simulink model "AMFC_Quad_New_01_VelEst_01"  (R2017b)
settings: Solver=ode45  StartTime=0.0  StopTime=360  RelTol=1e-3  EnableMultiTasking=on
InitFcn:
  | Cons_AMFC_Quad_New_01
values from neighbouring files (symbols this model uses):
  alpha_Slid = 0.01    [Cons_AMFC_Quad_New_01.m]    (also in Const_Vel_Est_02.m)
  B = 1e+0*eye(n)    [Cons_AMFC_Quad_New_01.m]    (also in Const_Vel_Est_02.m = 1e0*eye(n); constant_Rev01_4Agents_10.m = 1e0*eye(n); constant_Rev01_4Agents_9.m = 1e0*eye(n))
  BBT_inv = ((B'*B)^(-1))*B'    [Cons_AMFC_Quad_New_01.m]    (also in Const_Vel_Est_02.m; constant_Rev01_4Agents_10.m; constant_Rev01_4Agents_9.m)
  gamma_0 = 1e-0*diag([1e-3*ones(3,1);1e-0*ones(3,1)])    [Cons_AMFC_Quad_New_01.m]    (also in Const_Vel_Est_02.m = 1e-1*diag([1e-3*ones(3,1);1e-0*ones(3,1)]); constant_Rev01_4Agents_10.m = 1e+1*diag([1e-3*ones(3,1);1e-0*ones(3,1)]); constant_Rev01_4Agents_9.m = 1e+1*diag([1e-3*ones(6,1);1e-0*ones(6,1)]))
  gamma_1 = 1e+2*diag([1e-3*ones(3,1);1e-0*ones(3,1)])    [Cons_AMFC_Quad_New_01.m]    (also in Const_Vel_Est_02.m; constant_Rev01_4Agents_10.m = 1e+3*diag([1e-3*ones(3,1);1e0*ones(3,1)]); constant_Rev01_4Agents_9.m = 1e+3*diag([1e-3*ones(6,1);1e0*ones(6,1)]))
  ge = 9.81    [Cons_AMFC_Quad_New_01.m]
  J = 1.2416e-3 * diag([1 1 2])    [Cons_AMFC_Quad_New_01.m]    (also in Const_Vel_Est_02.m = 1.2416e-3 * diag([1 1 2],0); constant_Rev01_4Agents_10.m = 1.2416e-3 * diag([1 1 2],0); constant_Rev01_4Agents_9.m = 1.2416e-3 * diag([1 1 2],0))
  k1 = 10    [Cons_AMFC_Quad_New_01.m]    (also in Const_Vel_Est_02.m = 1; constant_Rev01_4Agents_10.m = 1; constant_Rev01_4Agents_9.m = 1)
  k1o = 1000    [Cons_AMFC_Quad_New_01.m]    (also in Const_Vel_Est_02.m)
  k2 = 0.1    [Cons_AMFC_Quad_New_01.m]    (also in Const_Vel_Est_02.m; constant_Rev01_4Agents_10.m = 1; constant_Rev01_4Agents_9.m = 1)
  k2o = 100    [Cons_AMFC_Quad_New_01.m]    (also in Const_Vel_Est_02.m)
  Ka = 0.01    [Cons_AMFC_Quad_New_01.m]    (also in Const_Vel_Est_02.m; constant_Rev01_4Agents_10.m; constant_Rev01_4Agents_9.m)
  Kd = 0.01    [Cons_AMFC_Quad_New_01.m]    (also in Const_Vel_Est_02.m; constant_Rev01_4Agents_10.m; constant_Rev01_4Agents_9.m)
  Kf = 1.0e-5    (= 1e-05)    [Cons_AMFC_Quad_New_01.m]    (also in Const_Vel_Est_02.m; constant_Rev01_4Agents_10.m; constant_Rev01_4Agents_9.m)
  Kt = 0.0435 * Kf    (= 4.35e-07)    [Cons_AMFC_Quad_New_01.m]    (also in Const_Vel_Est_02.m = 1e-07; constant_Rev01_4Agents_10.m = 1e-07; constant_Rev01_4Agents_9.m = 1e-07)
  L = 0.45    [Cons_AMFC_Quad_New_01.m]    (also in Const_Vel_Est_02.m = DN - AN; constant_Rev01_4Agents_10.m = DN - AN; constant_Rev01_4Agents_9.m = DN - AN)
  m = 6    [Cons_AMFC_Quad_New_01.m]    (also in Const_Vel_Est_02.m; Swing2d_01_const.m = 1)
  M = 2.95    [Cons_AMFC_Quad_New_01.m]    (also in Const_Vel_Est_02.m = 2; constant_Rev01_4Agents_10.m = 2; constant_Rev01_4Agents_9.m = 2)
  n = 6    [Cons_AMFC_Quad_New_01.m]    (also in Const_Vel_Est_02.m; constant_Rev01_4Agents_10.m; constant_Rev01_4Agents_9.m = 12)
  Q = 1e-1*eye(n)    [Cons_AMFC_Quad_New_01.m]    (also in Const_Vel_Est_02.m = 1e-2*eye(n); constant_Rev01_4Agents_10.m = 1e-3*eye(n); constant_Rev01_4Agents_9.m = 1e-3*eye(n))
  R = 1e+0*eye(m)    [Cons_AMFC_Quad_New_01.m]    (also in Const_Vel_Est_02.m = 1e-0*eye(n); constant_Rev01_4Agents_10.m = 1e-0*eye(n); constant_Rev01_4Agents_9.m = 1e-0*eye(n))
  rho_0 = 1e-1    (= 0.1)    [Cons_AMFC_Quad_New_01.m]    (also in Const_Vel_Est_02.m; constant_Rev01_4Agents_10.m = 10; constant_Rev01_4Agents_9.m = 10)
  rho_1 = 1e-0    (= 1)    [Cons_AMFC_Quad_New_01.m]    (also in Const_Vel_Est_02.m; constant_Rev01_4Agents_10.m = 0.1; constant_Rev01_4Agents_9.m = 0.1)
undefined symbols (not defined in the file or in its folder): sigbuilder_block
settings Model: Creator=hp  LastModifiedBy=ali.safaei
settings DataIOCC: LimitDataPoints=on  SaveFormat=Array
settings OptimizationCC: LifeSpan=inf
settings DebuggingCC: UnderspecifiedInitializationDetection=Classic  MergeDetectMultiDrivingBlocksExec=none  SolverPrmCheckMsg=warning  SFUnexpectedBacktrackingDiag=warning  SFNoUnconditionalDefaultTransitionDiag=warning  SFExecutionAtInitializationDiag=none
settings HardwareCC: ProdBitPerPointer=32  ProdBitPerSizeT=32  ProdBitPerPtrDiffT=32  ProdLargestAtomicFloat=None  ProdIntDivRoundTo=Undefined  ProdEndianess=Unspecified  ProdWordSize=32  ProdHWDeviceType=32-bit Generic
settings ModelReferenceCC: PropagateSignalLabelsOutOfModel=off
settings CodeAppCC: StateflowObjectComments=on
settings GRTTargetCC: TargetLangStandard=C89/C90 (ANSI)  GeneratePreprocessorConditionals=Disable all
settings ConfigComp: CovMetricSettings=dw  CovHtmlReporting=on  CovSaveCumulativeToWorkspaceVar=on  CovSaveSingleToWorkspaceVar=on  CovExternalEMLEnable=off

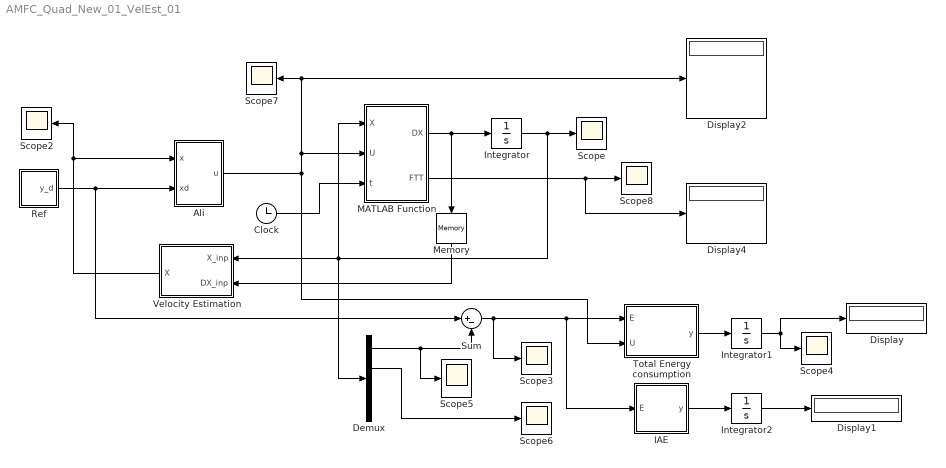
== system AMFC_Quad_New_01_VelEst_01 ==
  Ali : Subsystem
  Clock : Clock
  Demux : Demux
  Display{,1..2,4} (4 alike) : Display
  IAE : MATLAB Function  TreatAsAtomicUnit=on
  Integrator : Integrator  InitialCondition=zeros(12,1)
  Integrator1 : Integrator
  Integrator2 : Integrator
  MATLAB Function : MATLAB Function  TreatAsAtomicUnit=on
  Memory : Memory  InitialCondition=zeros(12,1)
  Ref : Subsystem
  Scope{,2..8} (8 alike) : Scope
  Sum : Sum  Inputs=|+-
  Total Energy consumption : MATLAB Function  TreatAsAtomicUnit=on
  Velocity Estimation : Subsystem
  wires:
  MATLAB Function/1(DX) -> Memory/1, Integrator/1
  Integrator/1 -> Scope/1, Demux/1, MATLAB Function/1(X), Velocity Estimation/1(X_inp)
  Integrator1/1 -> Display/1, Scope4/1
  Total Energy consumption/1(y) -> Integrator1/1
  Ref/1(y_d) -> Sum/1, Ali/2(xd)
  Integrator2/1 -> Display1/1
  Sum/1 -> Total Energy consumption/1(E), IAE/1(E), Scope3/1
  IAE/1(y) -> Integrator2/1
  Demux/1 -> Sum/2, Scope5/1
  Clock/1 -> MATLAB Function/3(t)
  Demux/2 -> Scope6/1
  Ali/1(u) -> Total Energy consumption/2(U), MATLAB Function/2(U), Display2/1, Scope7/1
  MATLAB Function/2(FTT) -> Scope8/1, Display4/1
  Velocity Estimation/1(X) -> Scope2/1, Ali/1(x)
  Memory/1 -> Velocity Estimation/2(DX_inp)

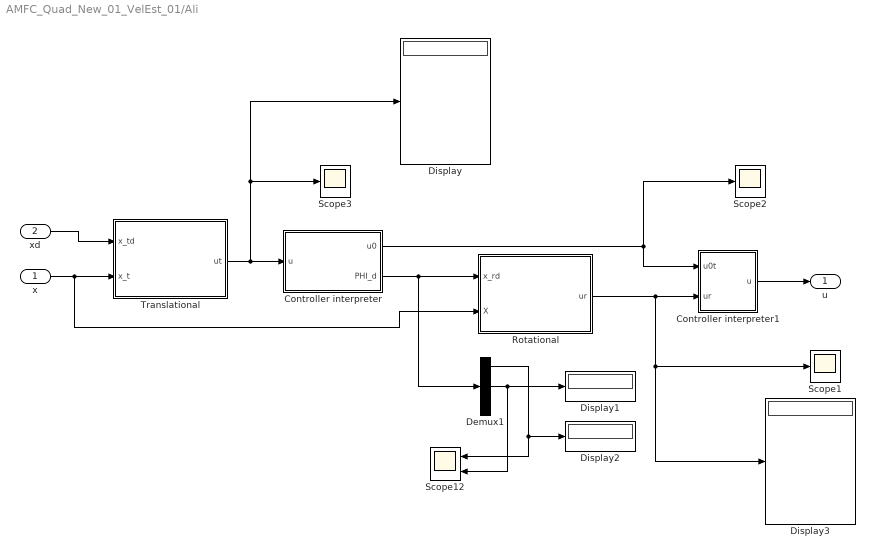
== system AMFC_Quad_New_01_VelEst_01/Ali ==
  x : Inport
  xd : Inport  Port=2
  Controller interpreter : MATLAB Function  TreatAsAtomicUnit=on
  Controller interpreter1 : MATLAB Function  TreatAsAtomicUnit=on
  Demux1 : Demux  Outputs=3
  Display{,1..3} (4 alike) : Display
  Rotational : Subsystem
  Scope1 : Scope
  Scope12 : Scope  NumInputPorts=2
  Scope2 : Scope
  Scope3 : Scope
  Translational : Subsystem
  u : Outport
  wires:
  Controller interpreter/2(PHI_d) -> Demux1/1, Rotational/1(x_rd)
  Rotational/1(ur) -> Display3/1, Scope1/1, Controller interpreter1/2(ur)
  Controller interpreter1/1(u) -> u/1
  Controller interpreter/1(u0) -> Scope2/1, Controller interpreter1/1(u0t)
  Demux1/2 -> Scope12/2, Display1/1
  Demux1/1 -> Display2/1, Scope12/1
  xd/1 -> Translational/1(x_td)
  x/1 -> Rotational/2(X), Translational/2(x_t)
  Translational/1(ut) -> Display/1, Scope3/1, Controller interpreter/1(u)

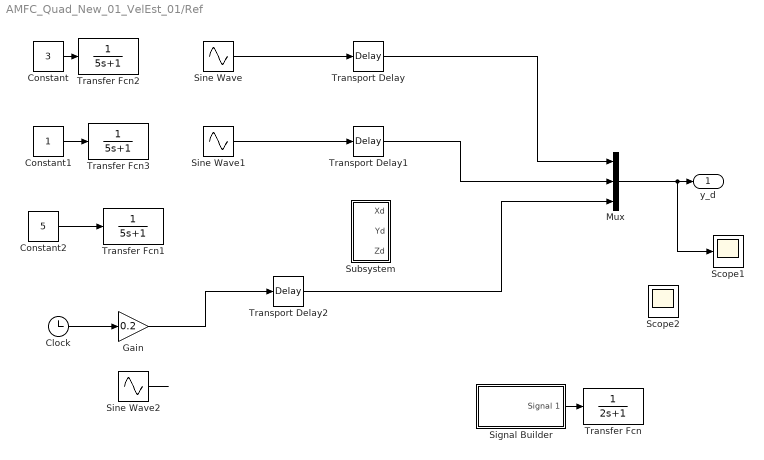
== system AMFC_Quad_New_01_VelEst_01/Ref ==
  Clock : Clock
  Constant : Constant  Value=3
  Constant1 : Constant
  Constant2 : Constant  Value=5
  Gain : Gain  Gain=0.2
  Mux : Mux  Inputs=3
  Scope1 : Scope
  Scope2 : Scope
  Signal Builder : Subsystem  Tag=STV Subsys  LoadFcn=sigbuilder_block('load');  StartFcn=sigbuilder_block('start');  StopFcn=sigbuilder_block('stop');  ClipboardFcn=sigbuilder_block('clipboard');  mask(Sigbuilder block){tuvar=[0:10]}
      mask help: Simulink:masks:SigbuilderBlock_MD
      mask init:
      | if ~strcmp(get_param(bdroot(gcbh),'SimulationStatus'),'stopped') tuvar = sigbuilder_block('maskInit'); end
      settings: CopyFcn=sigbuilder_block('copy');  DeleteFcn=sigbuilder_block('delete');  ModelCloseFcn=sigbuilder_block('modelClose');  PreSaveFcn=sigbuilder_block('preSave');  PauseFcn=sigbuilder_block('pause');  ContinueFcn=sigbuilder_block('continue');  NameChangeFcn=sigbuilder_block('namechange');  OpenFcn=sigbuilder_block('open',[437.25 117.75 550.5 394.5 ]);  CloseFcn=sigbuilder_block('close');
      mask Display: plot(0, 0, 100, 100,[2, 2, 32, 32, 2], [68, 8, 8, 68, 68],[32, 2], [38, 38], [32, 19, 2],[53, 60, 44], [32, 17, 17, 2],[16, 16, 31, 31]);txt = getActiveGroup(gcbh);text(2, 100, txt,'verticalAlignment', 'top');
  Sine Wave : Sin  Amplitude=10  Bias=-10  Frequency=0.2  Phase=pi/2  SampleTime=0
  Sine Wave1 : Sin  Amplitude=10  Frequency=0.2  SampleTime=0
  Sine Wave2 : Sin  Amplitude=2  Frequency=0.2  SampleTime=0
  Subsystem : Subsystem
  Transfer Fcn : TransferFcn  Denominator=[2 1]
  Transfer Fcn1 : TransferFcn  Denominator=[5 1]
  Transfer Fcn2 : TransferFcn  Denominator=[5 1]
  Transfer Fcn3 : TransferFcn  Denominator=[5 1]
  Transport Delay : TransportDelay  DelayTime=50
  Transport Delay1 : TransportDelay  DelayTime=50
  Transport Delay2 : TransportDelay  DelayTime=30
  y_d : Outport
  wires:
  Clock/1 -> Gain/1
  Signal Builder/1(Signal 1) -> Transfer Fcn/1
  Mux/1 -> Scope1/1, y_d/1
  Transport Delay/1 -> Mux/1
  Constant2/1 -> Transfer Fcn1/1
  Sine Wave1/1 -> Transport Delay1/1
  Sine Wave/1 -> Transport Delay/1
  Sine Wave2/1 -> ?
  Transport Delay1/1 -> Mux/2
  Constant/1 -> Transfer Fcn2/1
  Constant1/1 -> Transfer Fcn3/1
  Transport Delay2/1 -> Mux/3
  Gain/1 -> Transport Delay2/1

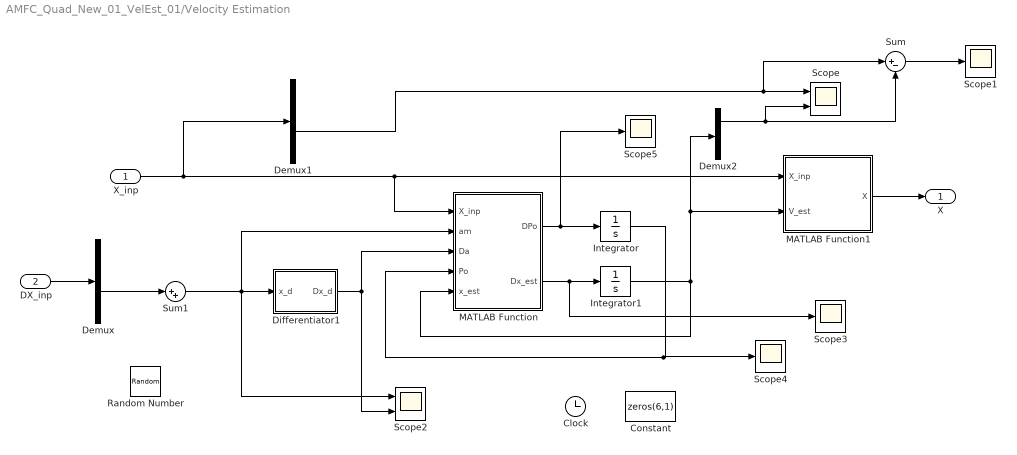
== system AMFC_Quad_New_01_VelEst_01/Velocity Estimation ==
  X_inp : Inport
  DX_inp : Inport  Port=2
  Clock : Clock
  Constant : Constant  Value=zeros(6,1)
  Demux : Demux
  Demux1 : Demux
  Demux2 : Demux  Outputs=2
  Differentiator1 : Subsystem
  Integrator : Integrator  InitialCondition=zeros(6)
  Integrator1 : Integrator  InitialCondition=zeros(6,1)
  MATLAB Function : MATLAB Function  TreatAsAtomicUnit=on
  MATLAB Function1 : MATLAB Function  TreatAsAtomicUnit=on
  Random Number : RandomNumber
  Scope : Scope  NumInputPorts=2
  Scope{1,3..5} (4 alike) : Scope
  Scope2 : Scope  NumInputPorts=2
  Sum : Sum  Inputs=|+-
  Sum1 : Sum  Inputs=|++
  X : Outport
  wires:
  DX_inp/1 -> Demux/1
  X_inp/1 -> Demux1/1, MATLAB Function/1(X_inp), MATLAB Function1/1(X_inp)
  MATLAB Function/1(DPo) -> Scope5/1, Integrator/1
  MATLAB Function/2(Dx_est) -> Integrator1/1, Scope3/1
  MATLAB Function1/1(X) -> X/1
  Differentiator1/1(Dx_d) -> Scope2/2, MATLAB Function/3(Da)
  Demux1/3 -> Sum/1, Scope/1
  Demux2/1 -> Sum/2, Scope/2
  Sum/1 -> Scope1/1
  Demux/3 -> Sum1/1
  Integrator1/1 -> MATLAB Function1/2(V_est), Demux2/1, MATLAB Function/5(x_est)
  Sum1/1 -> MATLAB Function/2(am), Differentiator1/1(x_d), Scope2/1
  Integrator/1 -> Scope4/1, MATLAB Function/4(Po)

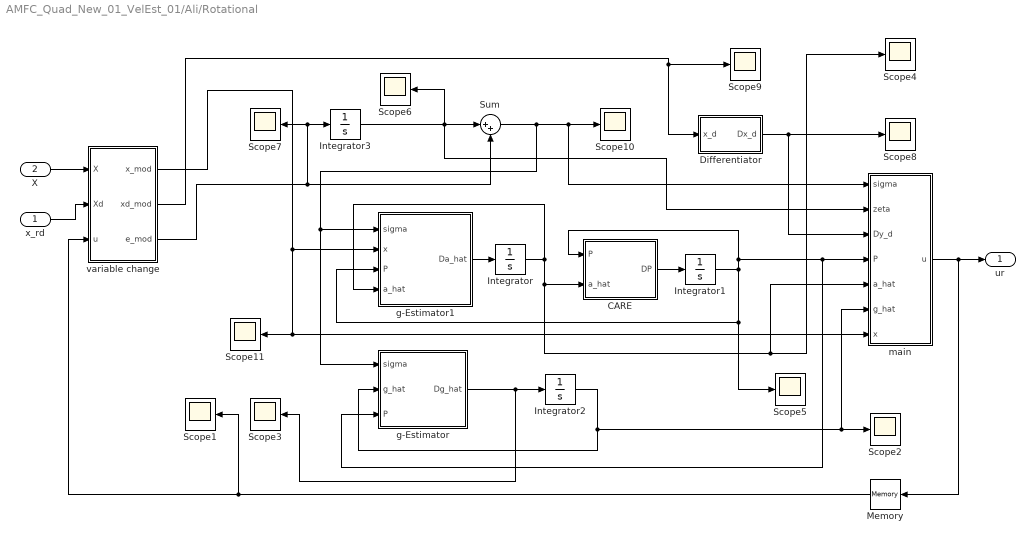
== system AMFC_Quad_New_01_VelEst_01/Ali/Rotational ==
  x_rd : Inport
  X : Inport  Port=2
  CARE : MATLAB Function  TreatAsAtomicUnit=on
  Differentiator : Subsystem
  Integrator : Integrator  InitialCondition=zeros(n)
  Integrator1 : Integrator  InitialCondition=eye(n)
  Integrator2 : Integrator  InitialCondition=zeros(n,1)
  Integrator3 : Integrator  InitialCondition=zeros(n,1)
  Memory : Memory  InitialCondition=zeros(m,1)
  Scope{1..11} (11 alike) : Scope
  Sum : Sum  Inputs=|++
  g-Estimator : MATLAB Function  TreatAsAtomicUnit=on
  g-Estimator1 : MATLAB Function  TreatAsAtomicUnit=on
  main : MATLAB Function  TreatAsAtomicUnit=on
  variable change : MATLAB Function  TreatAsAtomicUnit=on
  ur : Outport
  wires:
  x_rd/1 -> variable change/2(Xd)
  X/1 -> variable change/1(X)
  CARE/1(DP) -> Integrator1/1
  Sum/1 -> main/1(sigma), Scope10/1, g-Estimator/1(sigma), g-Estimator1/1(sigma)
  g-Estimator1/1(Da_hat) -> Integrator/1
  variable change/1(x_mod) -> Scope11/1, main/7(x), g-Estimator1/2(x)
  Integrator1/1 -> Scope5/1, g-Estimator1/3(P), CARE/1(P), g-Estimator/3(P), main/4(P)
  Integrator/1 -> g-Estimator1/4(a_hat), CARE/2(a_hat), main/5(a_hat), Scope4/1
  g-Estimator/1(Dg_hat) -> Scope3/1, Integrator2/1
  Differentiator/1(Dx_d) -> main/3(Dy_d), Scope8/1
  main/1(u) -> Memory/1, ur/1
  Integrator3/1 -> main/2(zeta), Scope6/1, Sum/1
  variable change/2(xd_mod) -> Scope9/1, Differentiator/1(x_d)
  variable change/3(e_mod) -> Sum/2, Scope7/1, Integrator3/1
  Memory/1 -> variable change/3(u), Scope1/1
  Integrator2/1 -> g-Estimator/2(g_hat), main/6(g_hat), Scope2/1

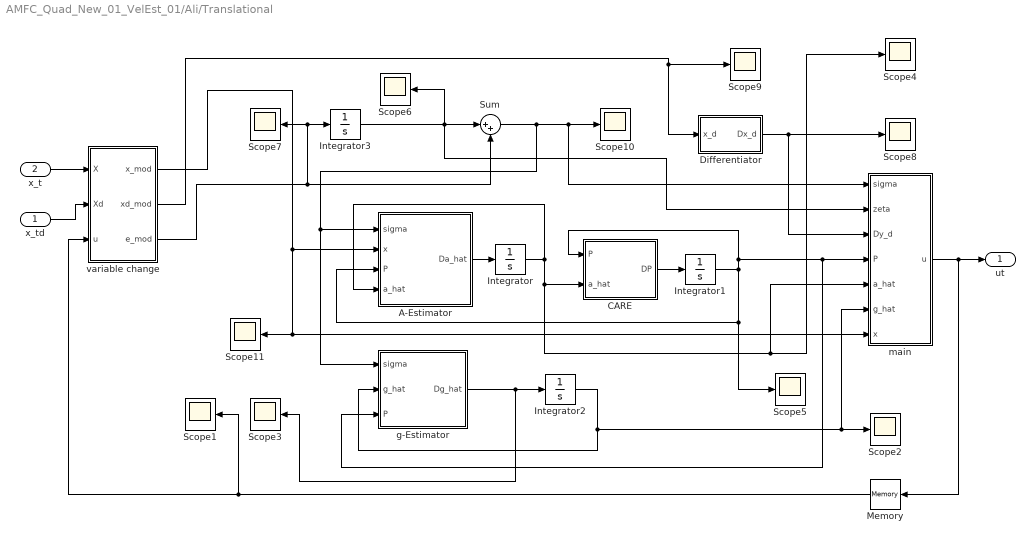
== system AMFC_Quad_New_01_VelEst_01/Ali/Translational ==
  x_td : Inport
  x_t : Inport  Port=2
  A-Estimator : MATLAB Function  TreatAsAtomicUnit=on
  CARE : MATLAB Function  TreatAsAtomicUnit=on
  Differentiator : Subsystem
  Integrator : Integrator  InitialCondition=zeros(n)
  Integrator1 : Integrator  InitialCondition=eye(n)
  Integrator2 : Integrator  InitialCondition=zeros(n,1)
  Integrator3 : Integrator  InitialCondition=zeros(n,1)
  Memory : Memory  InitialCondition=zeros(m,1)
  Scope{1..11} (11 alike) : Scope
  Sum : Sum  Inputs=|++
  g-Estimator : MATLAB Function  TreatAsAtomicUnit=on
  main : MATLAB Function  TreatAsAtomicUnit=on
  variable change : MATLAB Function  TreatAsAtomicUnit=on
  ut : Outport
  wires:
  Integrator2/1 -> Scope2/1, main/6(g_hat), g-Estimator/2(g_hat)
  Memory/1 -> Scope1/1, variable change/3(u)
  variable change/3(e_mod) -> Integrator3/1, Scope7/1, Sum/2
  variable change/2(xd_mod) -> Differentiator/1(x_d), Scope9/1
  Integrator3/1 -> Sum/1, Scope6/1, main/2(zeta)
  main/1(u) -> ut/1, Memory/1
  Differentiator/1(Dx_d) -> Scope8/1, main/3(Dy_d)
  g-Estimator/1(Dg_hat) -> Integrator2/1, Scope3/1
  Integrator/1 -> Scope4/1, main/5(a_hat), CARE/2(a_hat), A-Estimator/4(a_hat)
  Integrator1/1 -> main/4(P), g-Estimator/3(P), CARE/1(P), A-Estimator/3(P), Scope5/1
  variable change/1(x_mod) -> A-Estimator/2(x), main/7(x), Scope11/1
  A-Estimator/1(Da_hat) -> Integrator/1
  Sum/1 -> A-Estimator/1(sigma), g-Estimator/1(sigma), Scope10/1, main/1(sigma)
  CARE/1(DP) -> Integrator1/1
  x_td/1 -> variable change/2(Xd)
  x_t/1 -> variable change/1(X)

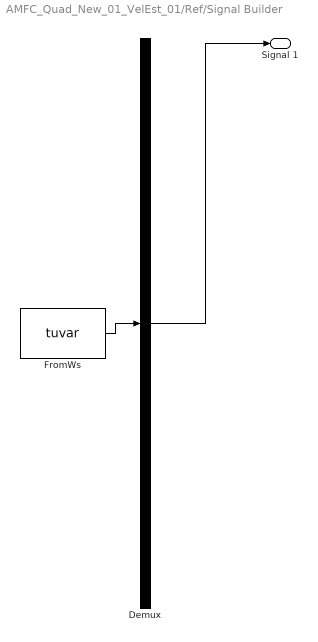
== system AMFC_Quad_New_01_VelEst_01/Ref/Signal Builder ==
  Demux : Demux  Tag=STV Demux  Outputs=1
  FromWs : FromWorkspace  Tag=STV FromWs  VariableName=tuvar  SampleTime=0
      SigBuilderData=|
      | common.afterFinalStr = 'Extrapolate'
      | common.sampleTime = 0
      | dataSet.timeRange = [0 100]
      | dataSet.name = 'Group 1'
      | sbobj.Groups.Name = 'Group 1'
      | sbobj.Groups.Signals.Name = 'Signal 1'
      | sbobj.Groups.Signals.XData = [0 20 20 50 50 100]
      | sbobj.Groups.Signals.YData = [0 0 2 2 0 0]
      | sbobj.Groups.TimeRange = [0 100]
  Signal 1 : Outport  Tag=STV Outport
  wires:
  Demux/1 -> Signal 1/1
  FromWs/1 -> Demux/1

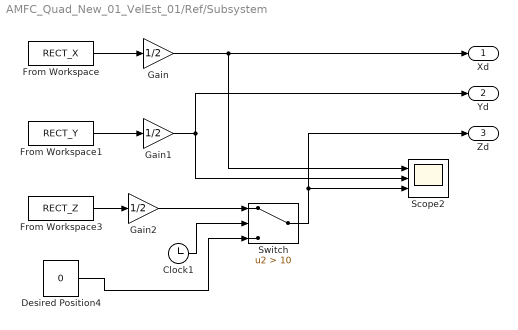
== system AMFC_Quad_New_01_VelEst_01/Ref/Subsystem ==
  Clock1 : Clock
  Desired Position4 : Constant  Value=0  VectorParams1D=off
  From Workspace : FromWorkspace  VariableName=RECT_X  SampleTime=0
  From Workspace1 : FromWorkspace  VariableName=RECT_Y  SampleTime=0
  From Workspace3 : FromWorkspace  VariableName=RECT_Z  SampleTime=0
  Gain : Gain  Gain=1/2
  Gain1 : Gain  Gain=1/2
  Gain2 : Gain  Gain=1/2
  Scope2 : Scope  NumInputPorts=3
  Switch : Switch  Criteria=u2 > Threshold  Threshold=10
  Xd : Outport
  Yd : Outport  Port=2
  Zd : Outport  Port=3
  wires:
  From Workspace/1 -> Gain/1
  From Workspace1/1 -> Gain1/1
  Clock1/1 -> Switch/2
  Switch/1 -> Zd/1, Scope2/3
  From Workspace3/1 -> Gain2/1
  Desired Position4/1 -> Switch/3
  Gain/1 -> Xd/1, Scope2/1
  Gain1/1 -> Yd/1, Scope2/2
  Gain2/1 -> Switch/1

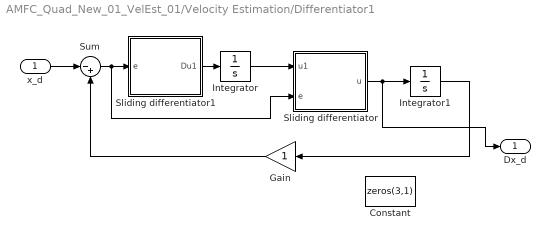
== system AMFC_Quad_New_01_VelEst_01/Velocity Estimation/Differentiator1 ==
  x_d : Inport
  Constant : Constant  Value=zeros(3,1)
  Gain : Gain
  Integrator : Integrator  InitialCondition=zeros(3,1)
  Integrator1 : Integrator  InitialCondition=zeros(3,1)
  Sliding differentiator : MATLAB Function  TreatAsAtomicUnit=on
  Sliding differentiator1 : MATLAB Function  TreatAsAtomicUnit=on
  Sum : Sum  Inputs=|-+
  Dx_d : Outport
  wires:
  Sliding differentiator1/1(Du1) -> Integrator/1
  Integrator/1 -> Sliding differentiator/1(u1)
  x_d/1 -> Sum/1
  Sum/1 -> Sliding differentiator/2(e), Sliding differentiator1/1(e)
  Integrator1/1 -> Gain/1
  Gain/1 -> Sum/2
  Sliding differentiator/1(u) -> Dx_d/1, Integrator1/1

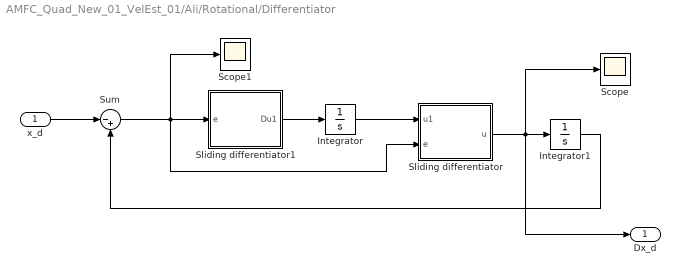
== system AMFC_Quad_New_01_VelEst_01/Ali/Rotational/Differentiator ==
  x_d : Inport
  Integrator : Integrator  InitialCondition=zeros(n,1)
  Integrator1 : Integrator  InitialCondition=zeros(n,1)
  Scope : Scope
  Scope1 : Scope
  Sliding differentiator : MATLAB Function  TreatAsAtomicUnit=on
  Sliding differentiator1 : MATLAB Function  TreatAsAtomicUnit=on
  Sum : Sum  Inputs=|-+
  Dx_d : Outport
  wires:
  Sliding differentiator/1(u) -> Scope/1, Integrator1/1, Dx_d/1
  Sliding differentiator1/1(Du1) -> Integrator/1
  Integrator/1 -> Sliding differentiator/1(u1)
  x_d/1 -> Sum/1
  Sum/1 -> Scope1/1, Sliding differentiator/2(e), Sliding differentiator1/1(e)
  Integrator1/1 -> Sum/2

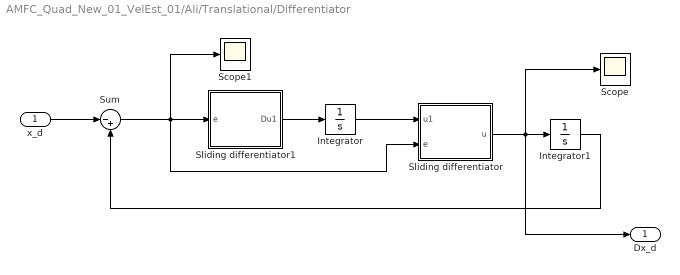
== system AMFC_Quad_New_01_VelEst_01/Ali/Translational/Differentiator ==
  x_d : Inport
  Integrator : Integrator  InitialCondition=zeros(n,1)
  Integrator1 : Integrator  InitialCondition=zeros(n,1)
  Scope : Scope
  Scope1 : Scope
  Sliding differentiator : MATLAB Function  TreatAsAtomicUnit=on
  Sliding differentiator1 : MATLAB Function  TreatAsAtomicUnit=on
  Sum : Sum  Inputs=|-+
  Dx_d : Outport
  wires:
  Integrator1/1 -> Sum/2
  Sum/1 -> Sliding differentiator1/1(e), Sliding differentiator/2(e), Scope1/1
  x_d/1 -> Sum/1
  Integrator/1 -> Sliding differentiator/1(u1)
  Sliding differentiator1/1(Du1) -> Integrator/1
  Sliding differentiator/1(u) -> Dx_d/1, Integrator1/1, Scope/1

== matlab function AMFC_Quad_New_01_VelEst_01/IAE ==
  data: E input; y output
function y = fcn(E)

Ea = abs(E(1:3));
% Qa = 1*eye(3);
y = sum(Ea); %Ea' * Qa * Ea;

end

== matlab function AMFC_Quad_New_01_VelEst_01/MATLAB Function ==
  data: X input; U input; t input; DX output; Kf parameter; Kt parameter; Kd parameter; Ka parameter; M parameter; J parameter; L parameter; ge parameter; FTT output
function [DX,FTT] = fcn(X,U,t,Kf,Kt,Kd,Ka,M,J,L,ge)

phi = X(4);
theta = X(5);
psi = X(6);

Rq = [cos(psi)*cos(theta) -sin(psi)*cos(phi)+cos(psi)*sin(theta)*sin(phi) sin(psi)*sin(phi)+cos(psi)*sin(theta)*cos(phi);
    sin(psi)*cos(theta) cos(psi)*cos(phi)+sin(psi)*sin(theta)*sin(phi) -cos(psi)*sin(phi)+sin(psi)*sin(theta)*cos(phi);
    -sin(theta) cos(theta)*sin(phi) cos(theta)*cos(phi)]; 

R_omega = [1 0 -sin(theta);
    0 cos(phi) cos(theta)*sin(phi);
    0 -sin(phi) cos(theta)*cos(phi)];

EXT_PRD = External_Product3(X(10:12),(J*X(10:12)));

F1 = Kf * U(1)^2;
F2 = Kf * U(2)^2;
F3 = Kf * U(3)^2;
F4 = Kf * U(4)^2;
  
FT = F1 + F2 + F3 + F4;
 
T1 = Kt * U(1)^2;
T2 = Kt * U(2)^2;
T3 = Kt * U(3)^2;
T4 = Kt * U(4)^2;
 
TT1 = L*(F3-F1);
TT2 = L*(F4-F2);
TT3 = (T1-T2+T3-T4);

FTT = Rq * [0;0;FT];
FTx = FTT(1);
FTy = FTT(2);
FTz = FTT(3);

DP = X(7:9);
DPHI = (R_omega)^(-1) * X(10:12); 
Dv = (1/M)*([FTx;FTy;FTz] - Kd*X(7:9) - M*[0;0;ge]) + Rq*(1*sin(1*t))*[0;0;1]; 
Dw = (J^(-1))*([TT1;TT2;TT3] - Ka*X(10:12) - EXT_PRD) + (1*sin(1*t)*[1;1;1]);

DX = [DP;DPHI;Dv;Dw];

end

== matlab function AMFC_Quad_New_01_VelEst_01/Velocity Estimation/MATLAB Function ==
  data: X_inp input; am input; DPo output; Da input; Dx_est output; Po input; x_est input
function [DPo,Dx_est] = fcn(X_inp,am,Da,Po,x_est)


phi = X_inp(4);
theta = X_inp(5);
psi = X_inp(6);

Rq = [cos(psi)*cos(theta) -sin(psi)*cos(phi)+cos(psi)*sin(theta)*sin(phi) sin(psi)*sin(phi)+cos(psi)*sin(theta)*cos(phi);
    sin(psi)*cos(theta) cos(psi)*cos(phi)+sin(psi)*sin(theta)*sin(phi) -cos(psi)*sin(phi)+sin(psi)*sin(theta)*cos(phi);
    -sin(theta) cos(theta)*sin(phi) cos(theta)*cos(phi)]; 

Ao = [zeros(3) Rq;
    zeros(3) zeros(3)];

Bo = [zeros(3);eye(3)];

Ho = [zeros(3) eye(3)];

Go = 1*eye(6);
Ro = 0.1*eye(3);
Qo = 1*eye(6);

uo = Da;
zo = am;

DPo = Ao*Po + Po*Ao' + Go*Qo*Go' - Po*Ho'*(Ro^-1)*Ho*Po;

Dx_est = Ao*x_est + Bo*uo + Po*Ho'*(Ro^-1)*(zo - Ho*x_est);

end

== matlab function AMFC_Quad_New_01_VelEst_01/Ali/Controller interpreter1 ==
  data: u output; u0t input; ur input; RM_1 parameter
function u = fcn(u0t,ur,RM_1)

y1 = ur(4);
y2 = ur(5);
y3 = ur(6);

Y = [u0t;y1;y2;y3];

u = RM_1*Y;
 
for i=1:4
    u(i) = sqrt(abs(u(i)));
end

end

== matlab function AMFC_Quad_New_01_VelEst_01/Ali/Rotational/CARE ==
  data: P input; a_hat input; B parameter; R parameter; DP output; Q parameter
function DP = fcn(P,a_hat,B,R,Q)

DP = a_hat*P + P*a_hat' - P*B*R*B'*P + 2*Q;

end

== matlab function AMFC_Quad_New_01_VelEst_01/Ali/Rotational/Differentiator/Sliding differentiator ==
  data: u output; u1 input; e input; n parameter; k1 parameter
function u = fcn(u1,e,n,k1)

b=k1;

ABS = zeros(n,1);
for i=1:n
    if e(i)>0
        ABS(i) = e(i);
    else
        ABS(i) = -e(i);
    end
end
SGN = e ./ (ABS + 0.01);

u = u1 - b*(ABS.^0.5).*SGN;

end

== matlab function AMFC_Quad_New_01_VelEst_01/Ali/Rotational/Differentiator/Sliding differentiator1 ==
  data: Du1 output; e input; n parameter; k2 parameter
function Du1 = fcn(e,n,k2)

a=k2;

ABS = zeros(n,1);
for i=1:n
    if e(i)>0
        ABS(i) = e(i);
    else
        ABS(i) = -e(i);
    end
end
SGN = e ./ (ABS + 0.01);

Du1 = - a*SGN;

end

== matlab function AMFC_Quad_New_01_VelEst_01/Ali/Rotational/g-Estimator ==
  data: sigma input; g_hat input; P input; rho_1 parameter; gamma_1 parameter; Dg_hat output
function Dg_hat = fcn(sigma,g_hat,P,rho_1,gamma_1)

Dg_hat = - gamma_1 * P * sigma - rho_1 * gamma_1 * g_hat;

end

== matlab function AMFC_Quad_New_01_VelEst_01/Ali/Rotational/g-Estimator1 ==
  data: sigma input; x input; P input; rho_0 parameter; gamma_0 parameter; Da_hat output; a_hat input
function Da_hat = fcn(sigma,x,P,rho_0,gamma_0,a_hat)

DVa_hat = - gamma_0 * P * diag(sigma) * (x - sigma) - rho_0 * gamma_0 * diag(a_hat);

Da_hat = diag(DVa_hat);

end

== matlab function AMFC_Quad_New_01_VelEst_01/Ali/Controller interpreter ==
  data: u0 output; PHI_d output size=3; u input
function [u0,PHI_d] = fcn(u)

u0 = sqrt((u(4)^2)+(u(5)^2)+(u(6)^2));

psi_d = 0;
phi_d = asin( min(max(((sin(psi_d)*u(4) - cos(psi_d)*u(5)) / (u0+1e-3)),-1),1) );
theta_d = atan( (cos(psi_d)*u(4) + sin(psi_d)*u(5)) / (u(6)+1e-3) );

PHI_d = [phi_d;theta_d;psi_d]; 

end

== matlab function AMFC_Quad_New_01_VelEst_01/Ali/Rotational/main ==
  data: sigma input; zeta input; u output; Dy_d input; R parameter; P input; a_hat input; B parameter; g_hat input; x input; Q parameter; BBT_inv parameter; n parameter
function u = fcn(sigma,zeta,Dy_d,R,P,a_hat,B,g_hat,x,Q,BBT_inv,n)

u1 = (1/2) * R * B' * P * sigma;
u2 = BBT_inv * (Dy_d - a_hat*x + (eye(n) + 2*(((P)^(-1)*Q)) + a_hat)*sigma - g_hat - zeta) - (3/4) * R * B' * P * sigma;

u = u1 + u2;

end

== matlab function AMFC_Quad_New_01_VelEst_01/Total Energy consumption ==
  data: E input; y output; U input
function y = fcn(E,U)

Ep = E(1:3);
Up = U(1:4);
Qe = 1*eye(3);
Re = 1*eye(4);
y = Ep' * Qe * Ep + Up' * Re * Up;

end

== matlab function AMFC_Quad_New_01_VelEst_01/Ali/Rotational/variable change ==
  data: X input; Xd input; x_mod output; u input; xd_mod output; e_mod output
function [x_mod,xd_mod,e_mod] = fcn(X,Xd,u)

x_mod = [X(4:6);X(10:12)];

xd_mod = [Xd;u(1:3)];

e_mod = xd_mod - x_mod;


end

== matlab function AMFC_Quad_New_01_VelEst_01/Velocity Estimation/Differentiator1/Sliding differentiator ==
  data: u output; u1 input; e input; k1o parameter; alpha_Slid parameter
function u = fcn(u1,e,k1o,alpha_Slid)

b=k1o;

ABS = abs(e);
SGN = e ./ (ABS + alpha_Slid);
u = u1 - b*((ABS.^0.5).*SGN); 

end

== matlab function AMFC_Quad_New_01_VelEst_01/Velocity Estimation/Differentiator1/Sliding differentiator1 ==
  data: Du1 output; e input; k2o parameter; alpha_Slid parameter
function Du1 = fcn(e,k2o,alpha_Slid)

a=k2o;

ABS = abs(e);
SGN = e ./ (ABS + alpha_Slid);
Du1 = - a*SGN;

end

== matlab function AMFC_Quad_New_01_VelEst_01/Velocity Estimation/MATLAB Function1 ==
  data: X_inp input; X output; V_est input
function X = fcn(X_inp,V_est)

X = [X_inp(1:6);V_est(1:3);X_inp(10:12)];

end

== matlab function AMFC_Quad_New_01_VelEst_01/Ali/Translational/CARE ==
  data: P input; a_hat input; B parameter; R parameter; DP output; Q parameter
function DP = fcn(P,a_hat,B,R,Q)

DP = a_hat*P + P*a_hat' - P*B*R*B'*P + 2*Q;

end

== matlab function AMFC_Quad_New_01_VelEst_01/Ali/Translational/Differentiator/Sliding differentiator ==
  data: u output; u1 input; e input; n parameter; k1 parameter
function u = fcn(u1,e,n,k1)

b=k1;

ABS = zeros(n,1);
for i=1:n
    if e(i)>0
        ABS(i) = e(i);
    else
        ABS(i) = -e(i);
    end
end
SGN = e ./ (ABS + 0.01);

u = u1 - b*(ABS.^0.5).*SGN;

end

== matlab function AMFC_Quad_New_01_VelEst_01/Ali/Translational/Differentiator/Sliding differentiator1 ==
  data: Du1 output; e input; n parameter; k2 parameter
function Du1 = fcn(e,n,k2)

a=k2;

ABS = zeros(n,1);
for i=1:n
    if e(i)>0
        ABS(i) = e(i);
    else
        ABS(i) = -e(i);
    end
end
SGN = e ./ (ABS + 0.01);

Du1 = - a*SGN;

end

== matlab function AMFC_Quad_New_01_VelEst_01/Ali/Translational/g-Estimator ==
  data: sigma input; g_hat input; P input; rho_1 parameter; gamma_1 parameter; Dg_hat output
function Dg_hat = fcn(sigma,g_hat,P,rho_1,gamma_1)

Dg_hat = - gamma_1 * P * sigma - rho_1 * gamma_1 * g_hat;

end

== matlab function AMFC_Quad_New_01_VelEst_01/Ali/Translational/A-Estimator ==
  data: sigma input; x input; P input; rho_0 parameter; gamma_0 parameter; Da_hat output; a_hat input
function Da_hat = fcn(sigma,x,P,rho_0,gamma_0,a_hat)

DVa_hat = - gamma_0 * P * diag(sigma) * (x - sigma) - rho_0 * gamma_0 * diag(a_hat);

Da_hat = diag(DVa_hat);

end

== matlab function AMFC_Quad_New_01_VelEst_01/Ali/Translational/main ==
  data: sigma input; zeta input; u output; Dy_d input; R parameter; P input; a_hat input; B parameter; g_hat input; x input; Q parameter; BBT_inv parameter; n parameter
function u = fcn(sigma,zeta,Dy_d,R,P,a_hat,B,g_hat,x,Q,BBT_inv,n)

u1 = (1/2) * R * B' * P * sigma;
u2 = BBT_inv * (Dy_d - a_hat*x + (eye(n) + 2*(((P)^(-1)*Q)) + a_hat)*sigma - g_hat - zeta) - (3/4) * R * B' * P * sigma;

u = u1 + u2;

end

== matlab function AMFC_Quad_New_01_VelEst_01/Ali/Translational/variable change ==
  data: X input; Xd input; x_mod output; u input; xd_mod output; e_mod output
function [x_mod,xd_mod,e_mod] = fcn(X,Xd,u)

x_mod = [X(1:3);X(7:9)];

xd_mod = [Xd;u(1:3)];

e_mod = xd_mod - x_mod;


end
